simulink model "SetSpeedIndicatorModel_withGUI"  (R2024a)
settings: Solver=VariableStepAuto  StartTime=0.0  StopTime=inf  RelTol=1e-3
settings Model: PacingRate=0.100000  Creator=tejesh  LastModifiedBy=darkh
settings DebuggingCC: UnderSpecifiedDimensionMsg=warning
settings ConfigComp: CovBoundaryAbsTol=1.0e-5

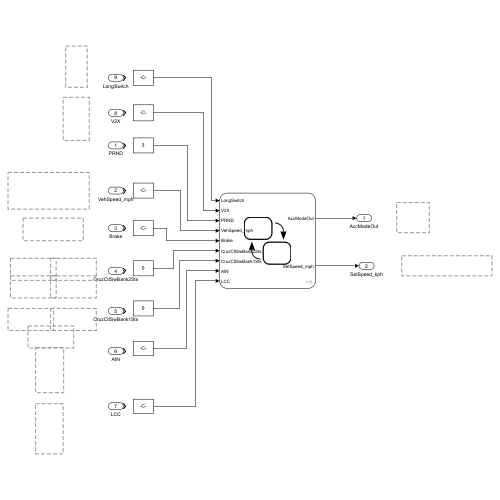
[thumbnail: Simulink's stored preview of the top-level diagram]
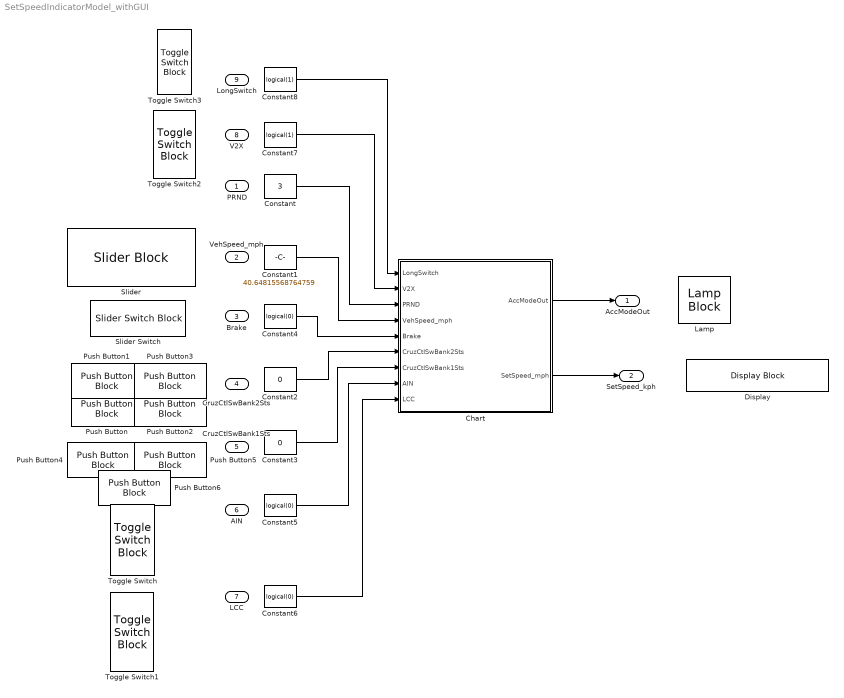
== system SetSpeedIndicatorModel_withGUI ==
  PRND : Inport
  VehSpeed_mph : Inport  Port=2
  Brake : Inport  Port=3
  CruzCtlSwBank2Sts : Inport  Port=4
  CruzCtlSwBank1Sts : Inport  Port=5
  AIN : Inport  Port=6
  LCC : Inport  Port=7
  V2X : Inport  Port=8
  LongSwitch : Inport  Port=9
  Chart : Stateflow chart  TreatAsAtomicUnit=on
      settings: PortSchema="{\"entries\":[{\"content\":{\"sides\":[{\"content\":{\"connectorIds\":[\"In8\",\"In9\",\"In1\",\"In2\",\"In3\",\"In4\",\"In5\",\"In6\",\"In7\"]},\"type\":\"ConnectorPlacement.EquallySpacedRectSide\",\"uuid\":\"e85dcfe6-766c-482d-aa65-e7bbb4e3e1c4\"},{\"content\":{\"connectorIds\":[\"Out1\",\"Out2\"],\"side\":\"RIGHT\"},\"type\":\"ConnectorPlacement.EquallySpacedRectSide\",\"uuid\":\"3867670f-d709-4b15-a3fa-6089a5f96600\"},{\"content\":{\"side\":\"TOP\"},\"type\":\"ConnectorPlacement.EquallySpacedRectSide\",\"uuid\":\"7701cee3-f3f2-4217-803b-6e8a4ec91dbe\"}]},\"type\":\"ConnectorPlacement.EquallySpacedConnector\",\"uuid\":\"080c218c-7887-4b4e-8a55-8cc53423266b\"}],\"packageUris\":[\"http://schema.mathworks.com/mf0/Connector/R2020b\"],\"version\":\"1.0\"}"
  Constant : Constant  Value=3
  Constant1 : Constant  Value=40.64815568764759
  Constant2 : Constant  Value=0
  Constant3 : Constant  Value=0
  Constant4 : Constant  Value=logical(0)  OutDataTypeStr=boolean
  Constant5 : Constant  Value=logical(0)  OutDataTypeStr=boolean
  Constant6 : Constant  Value=logical(0)  OutDataTypeStr=boolean
  Constant7 : Constant  Value=logical(1)  OutDataTypeStr=boolean
  Constant8 : Constant  Value=logical(1)  OutDataTypeStr=boolean
  Display : DisplayBlock  LabelPosition=Hide  Format=Integer  Transparency=1
  Lamp : LampBlock  LabelPosition=Hide
  Push Button : PushButtonBlock  ButtonText=SetShort  OffValue=0.000000
  Push Button1 : PushButtonBlock  ButtonText=ResumeShort  OnValue=2  OffValue=0.000000
  Push Button2 : PushButtonBlock  ButtonText=DecHigh  OnValue=3  OffValue=0.000000
  Push Button3 : PushButtonBlock  ButtonText=IncHigh  OnValue=4  OffValue=0.000000
  Push Button4 : PushButtonBlock  ButtonText=Off  OnValue=0  ButtonType=Latch  OffValue=2.000000
  Push Button5 : PushButtonBlock  ButtonText=On  ButtonType=Latch  OffValue=0.000000
  Push Button6 : PushButtonBlock  ButtonText=Cancel  OnValue=2  ButtonType=Latch  OffValue=1.000000
  Slider : SliderBlock
  Slider Switch : SliderSwitchBlock
      settings: Values={{'Off', 'On'}, [0 1]}
  Toggle Switch{,1..3} (4 alike) : ToggleSwitchBlock
      settings: Values={{'Off', 'On'}, [0 1]}
  AccModeOut : Outport
  SetSpeed_kph : Outport  Port=2
  wires:
  Chart/1(AccModeOut) -> AccModeOut/1
  Chart/2(SetSpeed_mph) -> SetSpeed_kph/1
  Constant/1 -> Chart/1(PRND)
  Constant1/1 -> Chart/2(VehSpeed_mph)
  Constant2/1 -> Chart/4(CruzCtlSwBank2Sts)
  Constant3/1 -> Chart/5(CruzCtlSwBank1Sts)
  Constant4/1 -> Chart/3(Brake)
  Constant5/1 -> Chart/6(AIN)
  Constant6/1 -> Chart/7(LCC)
  Constant7/1 -> Chart/9(V2X)
  Constant8/1 -> Chart/8(LongSwitch)

== stateflow chart SetSpeedIndicatorModel_withGUI/Chart ==
  state Armed
    entry:
    AccModeOut = AccModeType.ACC_Armed;
  state Off
    entry:
    AccModeOut = AccModeType.ACC_Off;
  state Engaged
    entry:
    AccModeOut = AccModeType.ACC_Engaged;
  Armed -> Off [order 3] : [PRND ~= PRNDType.D || CruzCtlSwBank1Sts == CruzCtlSwBank1Type.Off || ~V2X || ~ LongSwitch]
      | % Turn off if not in Drive OR CC Off button pressed OR V2X/Longitudinal Switch off
  (default) -> Off
  Engaged -> Armed [order 1] : [precondsOK(CruzCtlSwBank1Sts, VehSpeed_mph, Brake, AIN, LCC) == false]
      | % If any checks fail, go back to armed
  Off -> Armed : [CruzCtlSwBank1Sts == CruzCtlSwBank1Type.On && V2X && LongSwitch]
      | % Arm if CC On button pressed (with V2X and Longitudinal Switch ON)
  Armed -> Armed [order 1] : [CruzCtlSwBank2Sts == CruzCtlSwBank2Type.SetShort && precondsOK(CruzCtlSwBank1Sts, VehSpeed_mph, Brake, AIN, LCC)]
      | { SetSpeed_mph = VehSpeed_mph; hasValidSetSpeed = true; }
      | % Set speed for ACC
  Armed -> Engaged [order 2] : [CruzCtlSwBank2Sts == CruzCtlSwBank2Type.ResumeShort && precondsOK(CruzCtlSwBank1Sts, VehSpeed_mph, Brake, AIN, LCC) && hasValidSetSpeed]
      | % No change to SetSpeed, just engage
  Engaged -> Off [order 2] : [CruzCtlSwBank1Sts == CruzCtlSwBank1Type.Off]
      | % Turn off if CC Off button pressed
  Engaged -> Engaged [order 3] : [CruzCtlSwBank2Sts == CruzCtlSwBank2Type.SetShort && precondsOK(CruzCtlSwBank1Sts, VehSpeed_mph, Brake, AIN, LCC)]
      | { SetSpeed_mph = SetSpeed_mph - 1; }
      | % Decrease speed by 1
  Engaged -> Engaged [order 4] : [CruzCtlSwBank2Sts == CruzCtlSwBank2Type.ResumeShort && precondsOK(CruzCtlSwBank1Sts, VehSpeed_mph, Brake, AIN, LCC)]
      | { SetSpeed_mph = SetSpeed_mph + 1; }
      | % Increase speed by 1
  Engaged -> Engaged [order 6] : [CruzCtlSwBank2Sts == CruzCtlSwBank2Type.IncHigh && precondsOK(CruzCtlSwBank1Sts, VehSpeed_mph, Brake, AIN, LCC)]
      | { SetSpeed_mph = SetSpeed_mph + 5; }
      | % Increase speed by 5
  Engaged -> Engaged [order 5] : [CruzCtlSwBank2Sts == CruzCtlSwBank2Type.DecHigh && precondsOK(CruzCtlSwBank1Sts, VehSpeed_mph, Brake, AIN, LCC)]
      | { SetSpeed_mph = SetSpeed_mph - 5; }
      | % Decrease speed by 5
  data: SteeringInput function_input; Speed function_input; ok function_output; isBraking function_input; AIN_Active function_input; LCC_Active function_input; PRND input; VehSpeed_mph input; AccModeOut output; SetSpeed_mph output; hasValidSetSpeed local =false; Brake input; CruzCtlSwBank2Sts input; CruzCtlSwBank1Sts input; AIN input; LCC input; LongSwitch input; V2X input
  function ok = precondsOK(SteeringInput, Speed, isBraking, AIN_Active, LCC_Active):
    | function ok = precondsOK(SteeringInput, Speed, isBraking, AIN_Active, LCC_Active)
    | %#codegen
    | 
    |     % --- Determine allowable maximum speed ---
    |     % Default max speed (normal ACC)
    |     maxSpeed = 65;
    | 
    |     % If AIN is active, reduce to 55
    |     if AIN_Active
    |         maxSpeed = 55;
    |     end
    | 
    |     % If LCC is active, reduce even further to 35 (overrides AIN)
    |     if LCC_Active
    |         maxSpeed = 35;
    |     end
    | 
    |     % --- Evaluate Preconditions ---
    |     ok = (SteeringInput ~= CruzCtlSwBank1Type.Cancel) && ...
    |          (Speed >= 0 && Speed <= maxSpeed) && ...
    |          (isBraking == false);
    | end
